simulink subsystem "SensoresUS_016"  (R2023b)
settings: Solver=VariableStepAuto  StartTime=0.0  StopTime=10.0  RelTol=1e-3
libraries: arduinolib x2
settings Model: Creator=Enrique  LastModifiedBy=Enrique

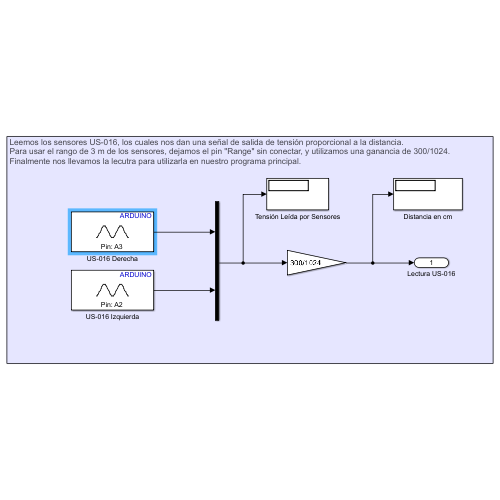
[thumbnail: Simulink's stored preview of the top-level diagram]
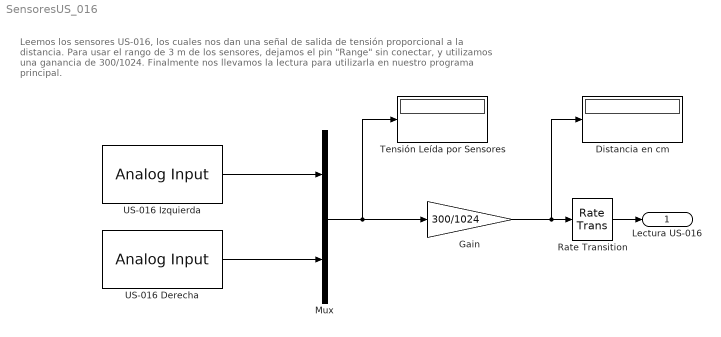
== system SensoresUS_016 ==
  note: Leemos los sensores US-016, los cuales nos dan una señal de salida de tensión proporcional a la distancia.
      | Para usar el rango de 3 m de los sensores, dejamos el pin "Range" sin conectar, y utilizamos una ganancia de 300/1024.
      | Finalmente nos llevamos la lectura para utilizarla en nuestro programa principal.
  Distancia en cm : Display
  Gain : Gain  Gain=300/1024
  Mux : Mux  Inputs=2
  Rate Transition : RateTransition  OutPortSampleTime=0.01
  Tensión Leída por Sensores : Display
  US-016 Derecha : arduinolib/Analog Input  pinNumber=3  ReadResultsOnly=off  ConversionTriggerSource=Software  ExternalTriggerType=uint32( 0 )  OutputDataType=uint16  EnableConversionCompleteNotify=off  EnableOuputStatus=off  SampleTime=0.05  blockPlatform=arduino
  US-016 Izquierda : arduinolib/Analog Input  pinNumber=2  ReadResultsOnly=off  ConversionTriggerSource=Software  ExternalTriggerType=uint32( 0 )  OutputDataType=uint16  EnableConversionCompleteNotify=off  EnableOuputStatus=off  SampleTime=0.05  blockPlatform=arduino
  Lectura US-016 : Outport
  wires:
  Mux/1 -> Gain/1, Tensión Leída por Sensores/1
  Gain/1 -> Distancia en cm/1, Rate Transition/1
  US-016 Derecha/1 -> Mux/2
  US-016 Izquierda/1 -> Mux/1
  Rate Transition/1 -> Lectura US-016/1
